simulink library "PB_Library_Master_Working"  (R2021a)
settings: Solver=VariableStepAuto  StartTime=0.0  StopTime=10.0  RelTol=1e-3
undefined symbols (not defined in the file): A_M, B_M, component_degradation_input, E0_M, f_sw, f_sw_M_aDF, flux_m_aDF, Fsw_M_aDF, insert, K_M, L_M_aDF, L_M_adf, P_Fe_Nom_aDF, Q_M, Q_rr, r_c, r_D, R_M, R_s_aDF, resistance_aDF, S_nom_aDF, SOC_Init_M, TFall_M_aDF, TRise_M_aDF, Trr_M_aDF, u_ce0, u_D0
libraries: $bdroot x76, Lib_Dyn_StateSpace_EMTAT x6, Lib_PF_BusLoadDC_TMATS x3, PB_Library_Master x3, simulink x3, TemperatureBlock x1
(part 3 of 5)

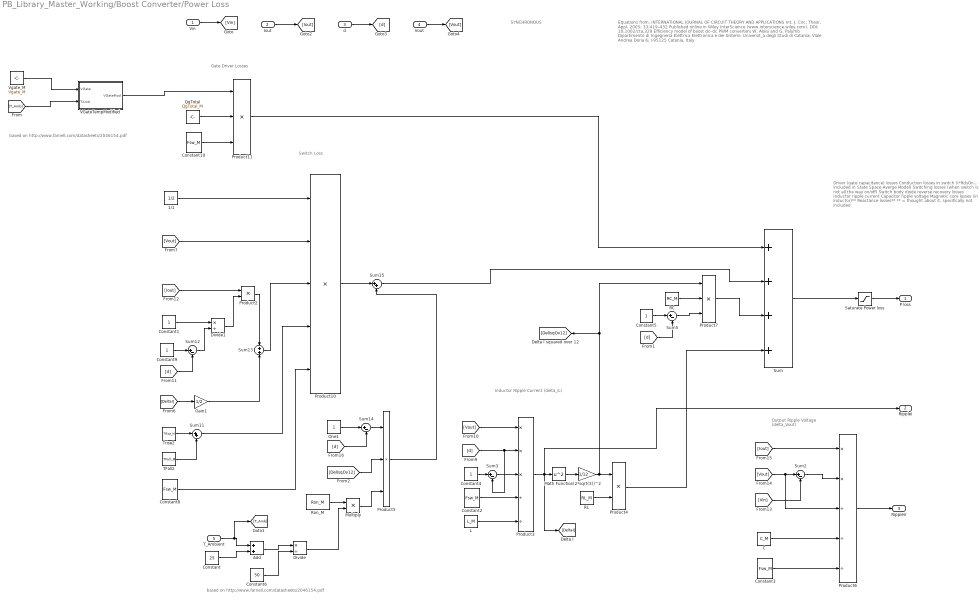
== system PB_Library_Master_Working/Boost Converter/Power Loss  ==
  note: Gate Driver Losses
  note: Output Ripple Voltage
      | (delta_Vout)
  note: Inductor Ripple Current
      | (delta_iL)
  note: Driver (gate capacitance) losses
      | Conduction losses in switch (I*RdsOn... included in State Space Averge Model)
      | Switching losses (when switch is not all the way on/off)
      | Switch body diode reverse recovery losses
      | Inductor ripple current
      | Capacitor ripple voltage
      | Magnetic core losses (in inductor)**
      | Reactance losses**
      | ** = thought about it, specifically not included
  note: SYNCHRONOUS
  note: Switch Loss
  note: Equations from:
      | INTERNATIONAL JOURNAL OF CIRCUIT THEORY AND APPLICATIONS
      | Int. J. Circ. Theor. Appl. 2005; 33:419–432
      | Published online in Wiley InterScience (www.interscience.wiley.com). DOI: 10.1002/cta.329
      | Efficiency model of boost dc–dc PWM converters
      | W. Aloisi and G. Palumb
      | Dipartimento di Ingegneria Elettrica Elettronica e dei Sistemi; Universit_a degli Studi di Catania;
      | Viale Andrea Doria 6; I-95125 Catania, Italy
  note: based on http://www.farnell.com/datasheets/2046154.pdf
  note: based on http://www.farnell.com/datasheets/2046154.pdf
  Vin : Inport
  Iout : Inport  Port=2
  d : Inport  Port=3
  Vout : Inport  Port=4
  "T_Ambient " : Inport  Port=5
  (2*sqrt(3))^2 : Gain  Gain=1/12
  1/1 : Constant  Value=1/2  VectorParams1D=off
  Add : Sum
  C : Constant  Value=C_M  VectorParams1D=off
  Constant : Constant  Value=25
  Constant{1,4..5,9} (4 alike) : Constant
  Constant{2..3,8,10} (4 alike) : Constant  Value=Fsw_M
  Constant6 : Constant  Value=50
  Divide : Product  Inputs=*/
  Divide1 : Product  Inputs=*/
  Gain1 : Gain  Gain=1/2
  L : Constant  Value=L_M  VectorParams1D=off
  Math Function : Math  Operator=square  SignedPower=on  SaturateOnIntegerOverflow=on
  Multiply : Product
  One1 : Constant  VectorParams1D=off
  Product10 : Product  Inputs=5
  Product11 : Product  Inputs=3
  Product2 : Product
  Product3 : Product  Inputs=***//
  Product4 : Product
  Product5 : Product  Inputs=3
  Product6 : Product  Inputs=**///
  Product7 : Product  Inputs=3
  QgTotal : Constant  Value=QgTotal_M  VectorParams1D=off
  RC : Constant  Value=RC_M  VectorParams1D=off
  RL : Constant  Value=RL_M  VectorParams1D=off
  Ron_M : Constant  Value=Ron_M
  Saturate Power loss : Saturate  UpperLimit=inf  LowerLimit=0
  Sum : Sum  Inputs=++++
  Sum11 : Sum  Inputs=|++
  Sum{2..3,5,12,14} (5 alike) : Sum  Inputs=|+-
  Sum13 : Sum
  Sum15 : Sum  Inputs=|++
  TFall2 : Constant  Value=TFall_M  VectorParams1D=off
  Trise2 : Constant  Value=TRise_M  VectorParams1D=off
  VGateTempModified : Subsystem
  "Vgate_M " : Constant  Value=Vgate_M
  " P loss" : Outport  VectorParamsAs1DForOutWhenUnconnected=off
  RippleI : Outport  Port=2  VectorParamsAs1DForOutWhenUnconnected=off
  RippleV : Outport  Port=3  VectorParamsAs1DForOutWhenUnconnected=off
  wires:
  VGateTempModified/1(VGateMod) -> Product11/1
  [T_Amb] -> VGateTempModified/2(TAmb)
  "Vgate_M "/1 -> VGateTempModified/1(VGate)
  Multiply/1 -> Product5/3
  Divide/1 -> Multiply/2
  Add/1 -> Divide/1
  Constant6/1 -> Divide/2
  Constant/1 -> Add/2
  "T_Ambient "/1 -> Add/1, [T_Amb]
  Sum15/1 -> Sum/2
  Product11/1 -> Sum/1
  Product7/1 -> Sum/3
  Product4/1 -> Sum/4
  QgTotal/1 -> Product11/2
  Constant10/1 -> Product11/3
  Product5/1 -> Sum15/2
  Product10/1 -> Sum15/1
  [DelIsqOv12] -> Product5/2
  Sum14/1 -> Product5/1
  Ron_M/1 -> Multiply/1
  One1/1 -> Sum14/1
  [d] -> Sum14/2
  Product6/1 -> RippleV/1
  Constant3/1 -> Product6/5
  C/1 -> Product6/4
  Sum2/1 -> Product6/2
  [Vin] -> Sum2/2
  [Vout] -> Sum2/1, Product6/3
  [Iout] -> Product6/1
  1/1/1 -> Product10/1
  [Vout] -> Product10/2
  Constant8/1 -> Product10/5
  Product2/1 -> Sum13/1
  Sum11/1 -> Product10/4
  Constant1/1 -> Divide1/1
  Trise2/1 -> Sum11/1
  TFall2/1 -> Sum11/2
  Divide1/1 -> Product2/2
  Sum12/1 -> Divide1/2
  Sum13/1 -> Product10/3
  Gain1/1 -> Sum13/2
  Constant9/1 -> Sum12/1
  [d] -> Sum12/2
  [DeltaI] -> Gain1/1
  [Iout] -> Product2/1
  Sum5/1 -> Product7/3
  [d] -> Sum5/2
  Constant5/1 -> Sum5/1
  Sum3/1 -> Product3/3
  Constant4/1 -> Sum3/1
  [Vout] -> Product3/1
  Constant2/1 -> Product3/4
  L/1 -> Product3/5
  Vout/1 -> [Vout]
  [d] -> Product3/2, Sum3/2
  d/1 -> [d]
  Iout/1 -> [Iout]
  Vin/1 -> [Vin]
  Sum/1 -> Saturate Power loss/1
  Saturate Power loss/1 -> " P loss"/1
  RL/1 -> Product4/2
  Product3/1 -> RippleI/1, Math Function/1, [DeltaI]
  (2*sqrt(3))^2/1 -> [DelIsqOv12], Product7/1, Product4/1
  Math Function/1 -> (2*sqrt(3))^2/1
  RC/1 -> Product7/2

== system PB_Library_Master_Working/Boost Converter/TempConv  ==
  Selected Input Units : Inport
  Unit Conversion : UnitConversion
  CelsiusOut : Outport  Unit=°C  VectorParamsAs1DForOutWhenUnconnected=off
  wires:
  Unit Conversion/1 -> CelsiusOut/1  "Celsius"
  Selected Input Units/1 -> Unit Conversion/1

== system PB_Library_Master_Working/Boost Converter Analytic/DC - DC Converter ==
  note: the aDF must decrease L_M
  note: Power B
  note: Current B
  note: Power B
  VIn : Inport
  x : Inport  Port=2
  d : Inport  Port=3
  dt : Inport  Port=4
  I_Demand : Inport  Port=5
  P loss : Inport  Port=6
  "T_Ambient " : Inport  Port=7
  " Dynamic State" : Subsystem  TreatAsAtomicUnit=on
  "1=dynamic, 0=static" : Display
  Add : Sum
  Bus Creator1 : BusCreator  Inputs=3
  Bus Creator3 : BusCreator  Inputs=3
  Bus Selector : BusSelector  OutputSignals=x,xdot,VB
  Constant : Constant  Value=[0, 1/C_M; -1/L_M, -(Ron_M+RC_M+RL_M)/L_M]  VectorParams1D=off
  Display : Display
  Divide : Product  Inputs=*/
  If : If
  MATLAB Function : MATLAB Function  TreatAsAtomicUnit=on
  Mux : Mux  Inputs=2
  Product3 : Product
  Steady State : Subsystem  TreatAsAtomicUnit=on
  Switch : Switch  Criteria=u2 ~= 0
  xdot : Constant  Value=zeros(2,1)  VectorParams1D=off
  VOut : Outport  VectorParamsAs1DForOutWhenUnconnected=off
  x_dot : Outport  Port=2  VectorParamsAs1DForOutWhenUnconnected=off
  x_new : Outport  Port=3  VectorParamsAs1DForOutWhenUnconnected=off
  I_Demanded : Outport  Port=4  VectorParamsAs1DForOutWhenUnconnected=off
  switchDyn : Outport  Port=5  VectorParamsAs1DForOutWhenUnconnected=off
  wires:
  "T_Ambient "/1 -> Steady State/3("T_Ambient "), Display/1
  Add/1 -> [PwrA]
  Mux/1 -> " Dynamic State"/2(u), Steady State/1(u)
  I_Demand/1 -> [IB], Mux/2
  [VA] -> Mux/1
  [x] -> x_new/1
  Bus Creator3/1 -> Switch/1
  Bus Selector/1 -> [x]  "<x>"
  Bus Selector/2 -> [xdot]  "<xdot>"
  Bus Selector/3 -> [VB]  "<VB>"
  xdot/1 -> Bus Creator1/2  "xdot"
  Steady State/2(VB) -> Bus Creator1/3  "VB"
  " Dynamic State"/1(xdot) -> Bus Creator3/2  "xdot"
  " Dynamic State"/2(VB) -> Bus Creator3/3  "VB"
  Switch/1 -> Bus Selector/1
  P loss/1 -> Add/2
  [PwrB] -> Add/1
  [xdot] -> x_dot/1
  d/1 -> " Dynamic State"/3(d), Steady State/2(d)
  x/1 -> " Dynamic State"/1(x), Bus Creator3/1  "x"
  Steady State/1(x) -> Bus Creator1/1  "x"
  dt/1 -> MATLAB Function/2(dt)
  If/2 -> Steady State/Action
  Constant/1 -> MATLAB Function/1(A1)
  If/1 -> " Dynamic State"/Action
  MATLAB Function/1(y) -> If/1, switchDyn/1, Switch/2, "1=dynamic, 0=static"/1
  [IA] -> I_Demanded/1
  [VA] -> Divide/2
  Divide/1 -> [IA]
  [PwrA] -> Divide/1
  [IB] -> Product3/2
  VIn/1 -> [VA]
  [VB] -> VOut/1  "V"
  Product3/1 -> [PwrB]
  [VB] -> Product3/1
  Bus Creator1/1 -> Switch/3

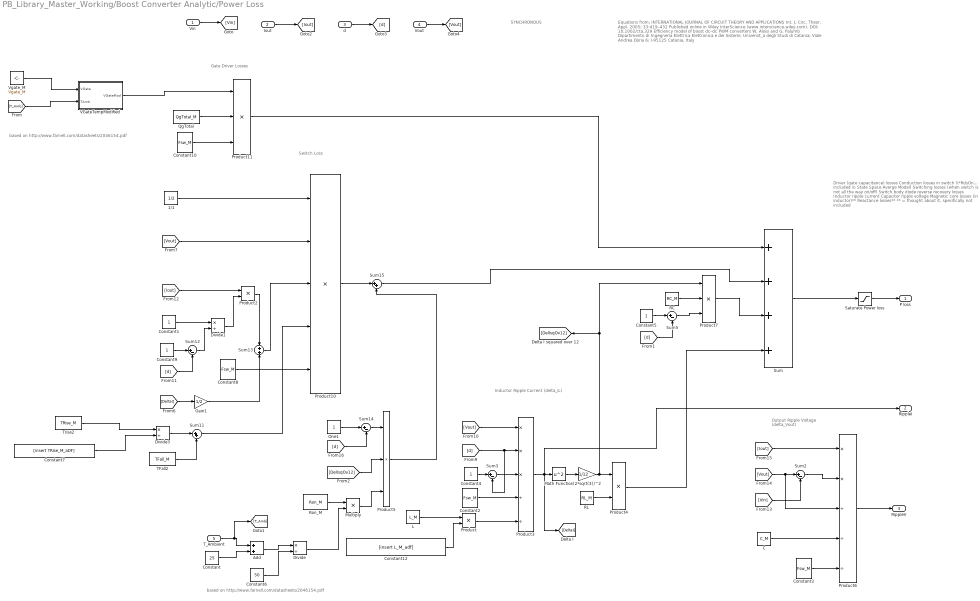
== system PB_Library_Master_Working/Boost Converter Analytic/Power Loss  ==
  note: Gate Driver Losses
  note: Output Ripple Voltage
      | (delta_Vout)
  note: Inductor Ripple Current
      | (delta_iL)
  note: Driver (gate capacitance) losses
      | Conduction losses in switch (I*RdsOn... included in State Space Averge Model)
      | Switching losses (when switch is not all the way on/off)
      | Switch body diode reverse recovery losses
      | Inductor ripple current
      | Capacitor ripple voltage
      | Magnetic core losses (in inductor)**
      | Reactance losses**
      | ** = thought about it, specifically not included
  note: SYNCHRONOUS
  note: Switch Loss
  note: Equations from:
      | INTERNATIONAL JOURNAL OF CIRCUIT THEORY AND APPLICATIONS
      | Int. J. Circ. Theor. Appl. 2005; 33:419–432
      | Published online in Wiley InterScience (www.interscience.wiley.com). DOI: 10.1002/cta.329
      | Efficiency model of boost dc–dc PWM converters
      | W. Aloisi and G. Palumb
      | Dipartimento di Ingegneria Elettrica Elettronica e dei Sistemi; Universit_a degli Studi di Catania;
      | Viale Andrea Doria 6; I-95125 Catania, Italy
  note: based on http://www.farnell.com/datasheets/2046154.pdf
  note: based on http://www.farnell.com/datasheets/2046154.pdf
  Vin : Inport
  Iout : Inport  Port=2
  d : Inport  Port=3
  Vout : Inport  Port=4
  "T_Ambient " : Inport  Port=5
  (2*sqrt(3))^2 : Gain  Gain=1/12
  1/1 : Constant  Value=1/2  VectorParams1D=off
  Add : Sum
  C : Constant  Value=C_M  VectorParams1D=off
  Constant : Constant  Value=25
  Constant{1,4..5,9} (4 alike) : Constant
  Constant{2..3,8,10} (4 alike) : Constant  Value=Fsw_M
  Constant12 : Constant  Value=[insert L_M_adf]
  Constant6 : Constant  Value=50
  Constant7 : Constant  Value=[insert TRise_M_aDF]
  Divide : Product  Inputs=*/
  Divide1 : Product  Inputs=*/
  Divide3 : Product  Inputs=*/
  Gain1 : Gain  Gain=1/2
  L : Constant  Value=L_M  VectorParams1D=off
  Math Function : Math  Operator=square  SignedPower=on  SaturateOnIntegerOverflow=on
  Multiply : Product
  One1 : Constant  VectorParams1D=off
  Product : Product
  Product10 : Product  Inputs=5
  Product11 : Product  Inputs=3
  Product2 : Product
  Product3 : Product  Inputs=***//
  Product4 : Product
  Product5 : Product  Inputs=3
  Product6 : Product  Inputs=**///
  Product7 : Product  Inputs=3
  QgTotal : Constant  Value=QgTotal_M  VectorParams1D=off
  RC : Constant  Value=RC_M  VectorParams1D=off
  RL : Constant  Value=RL_M  VectorParams1D=off
  Ron_M : Constant  Value=Ron_M
  Saturate Power loss : Saturate  UpperLimit=inf  LowerLimit=0
  Sum : Sum  Inputs=++++
  Sum11 : Sum  Inputs=|++
  Sum{2..3,5,12,14} (5 alike) : Sum  Inputs=|+-
  Sum13 : Sum
  Sum15 : Sum  Inputs=|++
  TFall2 : Constant  Value=TFall_M  VectorParams1D=off
  Trise2 : Constant  Value=TRise_M  VectorParams1D=off
  VGateTempModified : Subsystem
  "Vgate_M " : Constant  Value=Vgate_M
  " P loss" : Outport  VectorParamsAs1DForOutWhenUnconnected=off
  RippleI : Outport  Port=2  VectorParamsAs1DForOutWhenUnconnected=off
  RippleV : Outport  Port=3  VectorParamsAs1DForOutWhenUnconnected=off
  wires:
  VGateTempModified/1(VGateMod) -> Product11/1
  [T_Amb] -> VGateTempModified/2(TAmb)
  "Vgate_M "/1 -> VGateTempModified/1(VGate)
  Multiply/1 -> Product5/3
  Divide/1 -> Multiply/2
  Add/1 -> Divide/1
  Constant6/1 -> Divide/2
  Constant/1 -> Add/2
  "T_Ambient "/1 -> Add/1, [T_Amb]
  Sum15/1 -> Sum/2
  Product11/1 -> Sum/1
  Product7/1 -> Sum/3
  Product4/1 -> Sum/4
  QgTotal/1 -> Product11/2
  Product5/1 -> Sum15/2
  Product10/1 -> Sum15/1
  [DelIsqOv12] -> Product5/2
  Sum14/1 -> Product5/1
  One1/1 -> Sum14/1
  [d] -> Sum14/2
  Product6/1 -> RippleV/1
  C/1 -> Product6/4
  Sum2/1 -> Product6/2
  [Vin] -> Sum2/2
  [Vout] -> Sum2/1, Product6/3
  [Iout] -> Product6/1
  1/1/1 -> Product10/1
  [Vout] -> Product10/2
  Product2/1 -> Sum13/1
  Sum11/1 -> Product10/4
  Constant1/1 -> Divide1/1
  Divide1/1 -> Product2/2
  Sum12/1 -> Divide1/2
  Sum13/1 -> Product10/3
  Gain1/1 -> Sum13/2
  Constant9/1 -> Sum12/1
  [d] -> Sum12/2
  [DeltaI] -> Gain1/1
  [Iout] -> Product2/1
  Sum5/1 -> Product7/3
  [d] -> Sum5/2
  Constant5/1 -> Sum5/1
  Sum3/1 -> Product3/3
  Constant4/1 -> Sum3/1
  [Vout] -> Product3/1
  Vout/1 -> [Vout]
  [d] -> Product3/2, Sum3/2
  d/1 -> [d]
  Iout/1 -> [Iout]
  Vin/1 -> [Vin]
  Sum/1 -> Saturate Power loss/1
  Saturate Power loss/1 -> " P loss"/1
  RL/1 -> Product4/2
  Product3/1 -> RippleI/1, Math Function/1, [DeltaI]
  (2*sqrt(3))^2/1 -> [DelIsqOv12], Product7/1, Product4/1
  Math Function/1 -> (2*sqrt(3))^2/1
  RC/1 -> Product7/2
  Ron_M/1 -> Multiply/1
  Divide3/1 -> Sum11/1
  Trise2/1 -> Divide3/1
  Constant7/1 -> Divide3/2
  Constant10/1 -> Product11/3
  Constant8/1 -> Product10/5
  Constant2/1 -> Product3/4
  Constant3/1 -> Product6/5
  TFall2/1 -> Sum11/2
  Product/1 -> Product3/5
  L/1 -> Product/1
  Constant12/1 -> Product/2

== system PB_Library_Master_Working/Boost Converter Analytic/TempConv  ==
  Selected Input Units : Inport
  Unit Conversion : UnitConversion
  CelsiusOut : Outport  Unit=°C  VectorParamsAs1DForOutWhenUnconnected=off
  wires:
  Unit Conversion/1 -> CelsiusOut/1  "Celsius"
  Selected Input Units/1 -> Unit Conversion/1

== system PB_Library_Master_Working/Buck Converter/DC - DC Converter ==
  note: Power B
  note: Current B
  note: Power A
  NodeA : Inport
  IAg : Inport  Port=2
  x : Inport  Port=3
  d : Inport  Port=4
  dt : Inport  Port=5
  Iout : Inport  Port=6
  P loss : Inport  Port=7
  "T_Ambient " : Inport  Port=8
  " Dynamic State" : Subsystem  TreatAsAtomicUnit=on
  "1=dynamic, 0=static" : Display
  Add : Sum  Inputs=+-
  Bus Creator1 : BusCreator  Inputs=3
  Bus Creator3 : BusCreator  Inputs=3
  Bus Selector : BusSelector  OutputSignals=x,xdot,VB
  Constant : Constant  Value=[0, 1/C_M; -1/L_M, -(Ron_M+RC_M+RL_M)/L_M]  VectorParams1D=off
  Divide : Product  Commented=on  Inputs=*/
  Goto12 : Goto  Commented=on  GotoTag=IB
  Goto14 : From  Commented=on  GotoTag=PwrB
  Goto15 : From  Commented=on  GotoTag=VB
  Goto5 : From  Commented=on  GotoTag=IB
  If : If
  MATLAB Function : MATLAB Function  TreatAsAtomicUnit=on
  Mux : Mux  Inputs=2
  Negate : Gain  Commented=through  Gain=-1
  Product3 : Product
  Steady State : Subsystem  TreatAsAtomicUnit=on
  Switch : Switch  Criteria=u2 ~= 0
  xdot : Constant  Value=zeros(2,1)  VectorParams1D=off
  NodeB : Outport  VectorParamsAs1DForOutWhenUnconnected=off
  x_dot : Outport  Port=2  VectorParamsAs1DForOutWhenUnconnected=off
  x_new : Outport  Port=3  VectorParamsAs1DForOutWhenUnconnected=off
  PElec : Outport  Port=4  VectorParamsAs1DForOutWhenUnconnected=off
  IA : Outport  Port=5  VectorParamsAs1DForOutWhenUnconnected=off
  switchDyn : Outport  Port=6  VectorParamsAs1DForOutWhenUnconnected=off
  wires:
  "T_Ambient "/1 -> Steady State/3("T_Ambient ")
  Negate/1 -> [PwrB]
  Mux/1 -> " Dynamic State"/2(u), Steady State/1(u)
  Iout/1 -> Mux/2
  [VA] -> Mux/1
  [x] -> x_new/1
  Bus Creator3/1 -> Switch/1
  Bus Selector/1 -> [x]  "<x>"
  Bus Selector/2 -> [xdot]  "<xdot>"
  Bus Selector/3 -> [VB]  "<VB>"
  xdot/1 -> Bus Creator1/2  "xdot"
  Steady State/2(VB) -> Bus Creator1/3  "VB"
  " Dynamic State"/1(xdot) -> Bus Creator3/2  "xdot"
  " Dynamic State"/2(VB) -> Bus Creator3/3  "VB"
  Switch/1 -> Bus Selector/1
  Add/1 -> Negate/1
  P loss/1 -> Add/2
  [PwrA] -> Add/1
  [xdot] -> x_dot/1
  d/1 -> " Dynamic State"/3(d), Steady State/2(d)
  x/1 -> " Dynamic State"/1(x), Bus Creator3/1  "x"
  Steady State/1(x) -> Bus Creator1/1  "x"
  dt/1 -> MATLAB Function/2(dt)
  If/2 -> Steady State/Action
  Constant/1 -> MATLAB Function/1(A1)
  If/1 -> " Dynamic State"/Action
  MATLAB Function/1(y) -> If/1, switchDyn/1, Switch/2, "1=dynamic, 0=static"/1
  [IA] -> IA/1
  Goto5/1 -> ?  "I"
  IAg/1 -> [IA]
  Goto15/1 -> Divide/2
  Divide/1 -> Goto12/1
  Goto14/1 -> Divide/1
  [IA] -> Product3/2
  NodeA/1 -> [VA]
  [VB] -> NodeB/1  "V"
  Product3/1 -> [PwrA]
  [VA] -> Product3/1
  Bus Creator1/1 -> Switch/3
  [PwrB] -> PElec/1

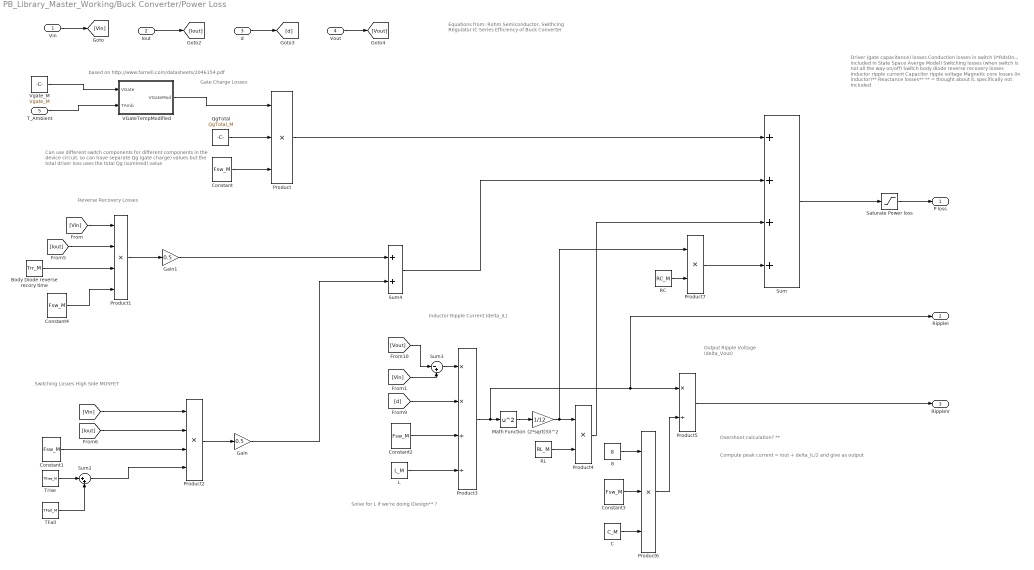
== system PB_Library_Master_Working/Buck Converter/Power Loss  ==
  note: based on http://www.farnell.com/datasheets/2046154.pdf
  note: Overshoot calculation? **
  note: Output Ripple Voltage
      | (delta_Vout)
  note: Inductor Ripple Current
      | (delta_iL)
  note: Reverse Recovery Losses
  note: Switching Losses High Side MOSFET
  note: Driver (gate capacitance) losses
      | Conduction losses in switch (I*RdsOn... included in State Space Averge Model)
      | Switching losses (when switch is not all the way on/off)
      | Switch body diode reverse recovery losses
      | Inductor ripple current
      | Capacitor ripple voltage
      | Magnetic core losses (in inductor)**
      | Reactance losses**
      | ** = thought about it, specifically not included
  note: Can use different switch components for different components in
      | the device circuit, so can have separate Qg (gate charge) values
      | but the total driver loss uses the total Qg (summed) value
  note: Gate Charge Losses
  note: Solve for L if we're doing iDesign** ?
  note: Compute peak current = Iout + delta_IL/2 and give as output
  note: Equations from:
      | Rohm Semiconductor, Swithcing Regulator IC Series
      | Efficiency of Buck Converter
  Vin : Inport
  Iout : Inport  Port=2
  d : Inport  Port=3
  Vout : Inport  Port=4
  "T_Ambient " : Inport  Port=5
  (2*sqrt(3))^2 : Gain  Gain=1/12
  8 : Constant  Value=8  VectorParams1D=off
  Body Diode reverse recory time : Constant  Value=Trr_M  VectorParams1D=off
  C : Constant  Value=C_M  VectorParams1D=off
  Constant{,1..4} (5 alike) : Constant  Value=Fsw_M
  Gain : Gain  Gain=0.5
  Gain1 : Gain  Gain=0.5
  L : Constant  Value=L_M  VectorParams1D=off
  Math Function : Math  Operator=square  SignedPower=on  SaturateOnIntegerOverflow=on
  Product : Product  Inputs=3
  Product1 : Product  Inputs=4
  Product2 : Product  Inputs=4
  Product3 : Product  Inputs=**//
  Product4 : Product
  Product5 : Product  Inputs=*/
  Product6 : Product  Inputs=3
  Product7 : Product
  QgTotal : Constant  Value=QgTotal_M  VectorParams1D=off
  RC : Constant  Value=RC_M  VectorParams1D=off
  RL : Constant  Value=RL_M  VectorParams1D=off
  Saturate Power loss : Saturate  UpperLimit=inf  LowerLimit=0
  Sum : Sum  Inputs=++++
  Sum2 : Sum  Inputs=|++
  Sum3 : Sum  Inputs=|-+
  Sum4 : Sum
  TFall : Constant  Value=TFall_M  VectorParams1D=off
  Trise : Constant  Value=TRise_M  VectorParams1D=off
  VGateTempModified : Subsystem
  Vgate_M : Constant  Value=Vgate_M
  " P loss" : Outport  VectorParamsAs1DForOutWhenUnconnected=off
  RippleI : Outport  Port=2  VectorParamsAs1DForOutWhenUnconnected=off
  RippleV : Outport  Port=3  VectorParamsAs1DForOutWhenUnconnected=off
  wires:
  VGateTempModified/1("VGateMod ") -> Product/1
  "T_Ambient "/1 -> VGateTempModified/2(TAmb)
  Vgate_M/1 -> VGateTempModified/1("VGate ")
  Gain1/1 -> Sum4/1
  Product1/1 -> Gain1/1
  Constant4/1 -> Product1/4
  Body Diode reverse recory time/1 -> Product1/3
  [Iout] -> Product1/2
  [Vin] -> Product1/1
  Gain/1 -> Sum4/2
  Product2/1 -> Gain/1
  Constant3/1 -> Product6/2
  Constant2/1 -> Product3/3
  Constant1/1 -> Product2/3
  Constant/1 -> Product/3
  [Vout] -> Sum3/1
  Vout/1 -> [Vout]
  [d] -> Product3/2
  d/1 -> [d]
  [Iout] -> Product2/2
  Iout/1 -> [Iout]
  [Vin] -> Sum3/2
  [Vin] -> Product2/1
  Vin/1 -> [Vin]
  Sum/1 -> Saturate Power loss/1
  Saturate Power loss/1 -> " P loss"/1
  QgTotal/1 -> Product/2
  Sum4/1 -> Sum/2
  Trise/1 -> Sum2/1
  TFall/1 -> Sum2/2
  Product/1 -> Sum/1
  Sum2/1 -> Product2/4
  Sum3/1 -> Product3/1
  L/1 -> Product3/4
  Product4/1 -> Sum/3
  RL/1 -> Product4/2
  Product3/1 -> Product5/1, RippleI/1, Math Function/1
  (2*sqrt(3))^2/1 -> Product7/1, Product4/1
  Math Function/1 -> (2*sqrt(3))^2/1
  Product6/1 -> Product5/2
  8/1 -> Product6/1
  C/1 -> Product6/3
  Product5/1 -> RippleV/1
  RC/1 -> Product7/2
  Product7/1 -> Sum/4

== system PB_Library_Master_Working/Buck Converter/TempConv  ==
  Selected Input Units : Inport
  Unit Conversion : UnitConversion
  CelsiusOut : Outport  Unit=°C  VectorParamsAs1DForOutWhenUnconnected=off
  wires:
  Unit Conversion/1 -> CelsiusOut/1  "Celsius"
  Selected Input Units/1 -> Unit Conversion/1

== system PB_Library_Master_Working/Buck Converter Analytic/DC - DC Converter ==
  note: Power A
  note: Current A
  note: Power B
  VIn : Inport
  x : Inport  Port=2
  d : Inport  Port=3
  dt : Inport  Port=4
  I_Demand : Inport  Port=5
  P loss : Inport  Port=6
  "T_Ambient " : Inport  Port=7
  " Dynamic State" : Subsystem  TreatAsAtomicUnit=on
  "1=dynamic, 0=static" : Display
  Add : Sum
  Bus Creator1 : BusCreator  Inputs=3
  Bus Creator3 : BusCreator  Inputs=3
  Bus Selector : BusSelector  OutputSignals=x,xdot,VB
  Constant : Constant  Value=[0, 1/C_M; -1/L_M, -(Ron_M+RC_M+RL_M)/L_M]  VectorParams1D=off
  Divide : Product  Inputs=*/
  If : If
  MATLAB Function : MATLAB Function  TreatAsAtomicUnit=on
  Mux : Mux  Inputs=2
  Product3 : Product
  Steady State : Subsystem  TreatAsAtomicUnit=on
  Switch : Switch  Criteria=u2 ~= 0
  xdot : Constant  Value=zeros(2,1)  VectorParams1D=off
  Vout : Outport  VectorParamsAs1DForOutWhenUnconnected=off
  x_dot : Outport  Port=2  VectorParamsAs1DForOutWhenUnconnected=off
  x_new : Outport  Port=3  VectorParamsAs1DForOutWhenUnconnected=off
  I_Demanded : Outport  Port=4  VectorParamsAs1DForOutWhenUnconnected=off
  switchDyn : Outport  Port=5  VectorParamsAs1DForOutWhenUnconnected=off
  wires:
  Bus Creator1/1 -> Switch/3
  [VB] -> Vout/1  "V"
  VIn/1 -> [VA]
  [IB] -> Product3/2
  [IA] -> I_Demanded/1
  MATLAB Function/1(y) -> "1=dynamic, 0=static"/1, Switch/2, switchDyn/1, If/1
  If/1 -> " Dynamic State"/Action
  Constant/1 -> MATLAB Function/1(A1)
  If/2 -> Steady State/Action
  dt/1 -> MATLAB Function/2(dt)
  Steady State/1(x) -> Bus Creator1/1  "x"
  x/1 -> Bus Creator3/1, " Dynamic State"/1(x)  "x"
  d/1 -> Steady State/2(d), " Dynamic State"/3(d)
  [xdot] -> x_dot/1
  P loss/1 -> Add/2
  Switch/1 -> Bus Selector/1
  " Dynamic State"/2(VB) -> Bus Creator3/3  "VB"
  " Dynamic State"/1(xdot) -> Bus Creator3/2  "xdot"
  Steady State/2(VB) -> Bus Creator1/3  "VB"
  xdot/1 -> Bus Creator1/2  "xdot"
  Bus Selector/3 -> [VB]  "<VB>"
  Bus Selector/2 -> [xdot]  "<xdot>"
  Bus Selector/1 -> [x]  "<x>"
  Bus Creator3/1 -> Switch/1
  [x] -> x_new/1
  [VA] -> Mux/1
  Mux/1 -> Steady State/1(u), " Dynamic State"/2(u)
  "T_Ambient "/1 -> Steady State/3("T_Ambient ")
  I_Demand/1 -> [IB], Mux/2
  [VB] -> Product3/1  "V"
  Product3/1 -> [PwrB]
  Divide/1 -> [IA]
  [PwrB] -> Add/1
  Add/1 -> [PwrA]
  [PwrA] -> Divide/1
  [VA] -> Divide/2

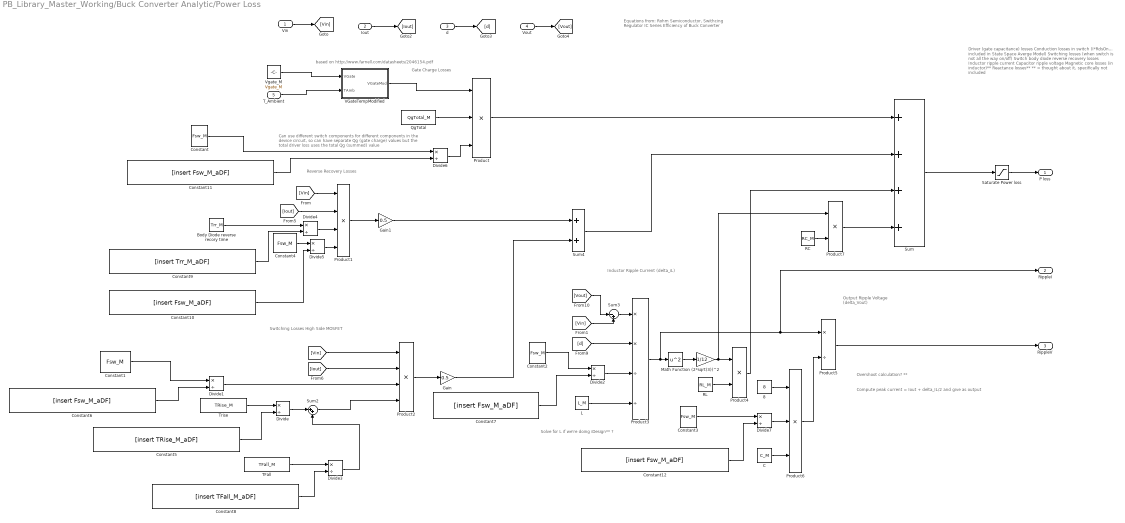
== system PB_Library_Master_Working/Buck Converter Analytic/Power Loss  ==
  note: Equations from:
      | Rohm Semiconductor, Swithcing Regulator IC Series
      | Efficiency of Buck Converter
  note: Compute peak current = Iout + delta_IL/2 and give as output
  note: Solve for L if we're doing iDesign** ?
  note: Gate Charge Losses
  note: Can use different switch components for different components in
      | the device circuit, so can have separate Qg (gate charge) values
      | but the total driver loss uses the total Qg (summed) value
  note: Driver (gate capacitance) losses
      | Conduction losses in switch (I*RdsOn... included in State Space Averge Model)
      | Switching losses (when switch is not all the way on/off)
      | Switch body diode reverse recovery losses
      | Inductor ripple current
      | Capacitor ripple voltage
      | Magnetic core losses (in inductor)**
      | Reactance losses**
      | ** = thought about it, specifically not included
  note: Switching Losses High Side MOSFET
  note: Reverse Recovery Losses
  note: Inductor Ripple Current
      | (delta_iL)
  note: Output Ripple Voltage
      | (delta_Vout)
  note: Overshoot calculation? **
  note: based on http://www.farnell.com/datasheets/2046154.pdf
  Vin : Inport
  Iout : Inport  Port=2
  d : Inport  Port=3
  Vout : Inport  Port=4
  "T_Ambient " : Inport  Port=5
  (2*sqrt(3))^2 : Gain  Gain=1/12
  8 : Constant  Value=8  VectorParams1D=off
  Body Diode reverse recory time : Constant  Value=Trr_M  VectorParams1D=off
  C : Constant  Value=C_M  VectorParams1D=off
  Constant{,1..4} (5 alike) : Constant  Value=Fsw_M
  Constant{6..7,10..12} (5 alike) : Constant  Value=[insert Fsw_M_aDF]
  Constant5 : Constant  Value=[insert TRise_M_aDF]
  Constant8 : Constant  Value=[insert TFall_M_aDF]
  Constant9 : Constant  Value=[insert Trr_M_aDF]
  Divide{,1..7} (8 alike) : Product  Inputs=*/
  Gain : Gain  Gain=0.5
  Gain1 : Gain  Gain=0.5
  L : Constant  Value=L_M  VectorParams1D=off
  Math Function : Math  Operator=square  SignedPower=on  SaturateOnIntegerOverflow=on
  Product : Product  Inputs=3
  Product1 : Product  Inputs=4
  Product2 : Product  Inputs=4
  Product3 : Product  Inputs=**//
  Product4 : Product
  Product5 : Product  Inputs=*/
  Product6 : Product  Inputs=3
  Product7 : Product
  QgTotal : Constant  Value=QgTotal_M  VectorParams1D=off
  RC : Constant  Value=RC_M  VectorParams1D=off
  RL : Constant  Value=RL_M  VectorParams1D=off
  Saturate Power loss : Saturate  UpperLimit=inf  LowerLimit=0
  Sum : Sum  Inputs=++++
  Sum2 : Sum  Inputs=|++
  Sum3 : Sum  Inputs=|-+
  Sum4 : Sum
  TFall : Constant  Value=TFall_M  VectorParams1D=off
  Trise : Constant  Value=TRise_M  VectorParams1D=off
  VGateTempModified : Subsystem
  Vgate_M : Constant  Value=Vgate_M
  " P loss" : Outport  VectorParamsAs1DForOutWhenUnconnected=off
  RippleI : Outport  Port=2  VectorParamsAs1DForOutWhenUnconnected=off
  RippleV : Outport  Port=3  VectorParamsAs1DForOutWhenUnconnected=off
  wires:
  Product7/1 -> Sum/4
  RC/1 -> Product7/2
  Product5/1 -> RippleV/1
  C/1 -> Product6/3
  8/1 -> Product6/1
  Product6/1 -> Product5/2
  Math Function/1 -> (2*sqrt(3))^2/1
  (2*sqrt(3))^2/1 -> Product4/1, Product7/1
  Product3/1 -> Math Function/1, RippleI/1, Product5/1
  RL/1 -> Product4/2
  Product4/1 -> Sum/3
  L/1 -> Product3/4
  Sum3/1 -> Product3/1
  Sum2/1 -> Product2/4
  Product/1 -> Sum/1
  Sum4/1 -> Sum/2
  QgTotal/1 -> Product/2
  Saturate Power loss/1 -> " P loss"/1
  Sum/1 -> Saturate Power loss/1
  Vin/1 -> [Vin]
  [Vin] -> Product2/1
  [Vin] -> Sum3/2
  Iout/1 -> [Iout]
  [Iout] -> Product2/2
  d/1 -> [d]
  [d] -> Product3/2
  Vout/1 -> [Vout]
  [Vout] -> Sum3/1
  Product2/1 -> Gain/1
  Gain/1 -> Sum4/2
  [Vin] -> Product1/1
  [Iout] -> Product1/2
  Product1/1 -> Gain1/1
  Gain1/1 -> Sum4/1
  Vgate_M/1 -> VGateTempModified/1("VGate ")
  "T_Ambient "/1 -> VGateTempModified/2(TAmb)
  VGateTempModified/1("VGateMod ") -> Product/1
  Divide/1 -> Sum2/1
  Trise/1 -> Divide/1
  Constant5/1 -> Divide/2
  Divide1/1 -> Product2/3
  Constant1/1 -> Divide1/1
  Constant6/1 -> Divide1/2
  Divide2/1 -> Product3/3
  Constant2/1 -> Divide2/1
  Constant7/1 -> Divide2/2
  Divide3/1 -> Sum2/2
  TFall/1 -> Divide3/1
  Constant8/1 -> Divide3/2
  Divide4/1 -> Product1/3
  Body Diode reverse recory time/1 -> Divide4/1
  Constant9/1 -> Divide4/2
  Divide5/1 -> Product1/4
  Constant4/1 -> Divide5/1
  Constant10/1 -> Divide5/2
  Divide6/1 -> Product/3
  Constant/1 -> Divide6/1
  Constant11/1 -> Divide6/2
  Divide7/1 -> Product6/2
  Constant3/1 -> Divide7/1
  Constant12/1 -> Divide7/2

== system PB_Library_Master_Working/Buck Converter Analytic/TempConv  ==
  Selected Input Units : Inport
  Unit Conversion : UnitConversion
  CelsiusOut : Outport  Unit=°C  VectorParamsAs1DForOutWhenUnconnected=off
  wires:
  Selected Input Units/1 -> Unit Conversion/1
  Unit Conversion/1 -> CelsiusOut/1  "Celsius"

== system PB_Library_Master_Working/Electrothermal_Battery_Model/Battery Core (w// Q) ==
  it_base : Inport
  IgIn : Inport  Port=2
  Tavg : Inport  Port=3
  BatteryCore : Subsystem
  Constant1 : Constant  Value=SOC_Init_M
  Vout : Outport  VectorParamsAs1DForOutWhenUnconnected=off
  SOC : Outport  Port=2  VectorParamsAs1DForOutWhenUnconnected=off
  it : Outport  Port=3  VectorParamsAs1DForOutWhenUnconnected=off
  Heat_Generated : Outport  Port=4  VectorParamsAs1DForOutWhenUnconnected=off
  wires:
  IgIn/1 -> BatteryCore/3("Battery Current (A) ")
  Constant1/1 -> BatteryCore/1("SOC Init (%) ")
  Tavg/1 -> BatteryCore/4("Tavg ")
  it_base/1 -> BatteryCore/2("it base (Ah) ")
  BatteryCore/2(it (Ah)) -> it/1
  BatteryCore/1(Battery Voltage (V)) -> Vout/1
  BatteryCore/3(SOC (%)) -> SOC/1
  BatteryCore/4(Heat_Generated) -> Heat_Generated/1

== system PB_Library_Master_Working/Electrothermal_Battery_Model/TempConv  ==
  Selected Input Units : Inport
  Unit Conversion : UnitConversion
  CelsiusOut : Outport  Unit=°C  VectorParamsAs1DForOutWhenUnconnected=off
  wires:
  Unit Conversion/1 -> CelsiusOut/1  "Celsius"
  Selected Input Units/1 -> Unit Conversion/1

== system PB_Library_Master_Working/Electrothermal_Battery_Model/it_Dot = f(i) ==
  i : Inport
  Convert As/s to Ah/s : Gain  Gain=1/3600
  it_Dot : Outport  VectorParamsAs1DForOutWhenUnconnected=off
  wires:
  Convert As/s to Ah/s/1 -> it_Dot/1
  i/1 -> Convert As/s to Ah/s/1

== system PB_Library_Master_Working/Electrothermal_Battery_Model_Analytic/Battery Core (w// Q) ==
  it_base : Inport
  I_Demand : Inport  Port=2
  Tavg : Inport  Port=3
  BatteryCore : Subsystem
  Constant1 : Constant  Value=SOC_Init_M
  Vout : Outport  VectorParamsAs1DForOutWhenUnconnected=off
  SOC : Outport  Port=2  VectorParamsAs1DForOutWhenUnconnected=off
  it : Outport  Port=3  VectorParamsAs1DForOutWhenUnconnected=off
  Heat_Generated : Outport  Port=4  VectorParamsAs1DForOutWhenUnconnected=off
  wires:
  I_Demand/1 -> BatteryCore/3("Battery Current (A) ")
  Constant1/1 -> BatteryCore/1("SOC Init (%) ")
  Tavg/1 -> BatteryCore/4("Tavg ")
  it_base/1 -> BatteryCore/2("it base (Ah) ")
  BatteryCore/2(it (Ah)) -> it/1
  BatteryCore/1(Battery Voltage (V)) -> Vout/1
  BatteryCore/3(SOC (%)) -> SOC/1
  BatteryCore/4(Heat_Generated) -> Heat_Generated/1

== system PB_Library_Master_Working/Electrothermal_Battery_Model_Analytic/it_Dot = f(i) ==
  i : Inport
  Convert As/s to Ah/s : Gain  Gain=1/3600
  it_Dot : Outport  VectorParamsAs1DForOutWhenUnconnected=off
  wires:
  Convert As/s to Ah/s/1 -> it_Dot/1
  i/1 -> Convert As/s to Ah/s/1

== system PB_Library_Master_Working/Generator/Copper Losses ==
  Iq : Inport
  Id1 : Inport  Port=2
  Constant : Constant  Value=[insert R_s_aDF]
  Constant1 : Constant  Value=[insert R_s_aDF]
  Divide : Product  Inputs=/*
  Divide1 : Product  Inputs=*/
  Gain1 : Gain  Gain=R_s
  Gain2 : Gain  Gain=R_s
  Square1 : Math  Operator=square  SignedPower=on  SaturateOnIntegerOverflow=on
  Square2 : Math  Operator=square  SignedPower=on  SaturateOnIntegerOverflow=on
  Sum : Sum
  P_Cu : Outport  VectorParamsAs1DForOutWhenUnconnected=off
  wires:
  Sum/1 -> P_Cu/1
  Square1/1 -> Gain1/1
  Iq/1 -> Square1/1
  Divide1/1 -> Sum/2
  Divide/1 -> Sum/1
  Gain1/1 -> Divide1/1
  Constant1/1 -> Divide1/2
  Gain2/1 -> Divide/2
  Id1/1 -> Square2/1
  Square2/1 -> Gain2/1
  Constant/1 -> Divide/1

== system PB_Library_Master_Working/Generator/Field Weakening and d current  ==
  note: Needs: S_n,flux_m,L_s
  S : Inport
  Constant : Constant  Value=flux_m
  Constant1 : Constant  Value=S_nom
  Constant2 : Constant  Value=[insert flux_m_aDF]
  Divide : Product  Inputs=*/
  Gain : Gain  Gain=1/L_s
  Product : Product
  Product1 : Product
  Subtract : Sum  Inputs=+-
  Switch : Switch  Criteria=u2 > Threshold  Threshold=S_nom
  flux_s : Outport  VectorParamsAs1DForOutWhenUnconnected=off
  Id : Outport  Port=2  VectorParamsAs1DForOutWhenUnconnected=off
  wires:
  S/1 -> Divide/2, Switch/2
  Product/1 -> Switch/1
  Divide/1 -> Product/2
  Switch/1 -> Subtract/1, flux_s/1
  Subtract/1 -> Gain/1
  Gain/1 -> Id/1
  Product1/1 -> Switch/3, Product/1, Subtract/2
  Constant/1 -> Product1/1
  Constant2/1 -> Product1/2
  Constant1/1 -> Divide/1

== system PB_Library_Master_Working/Generator/I_rms (Actual) ==
  note: I_RMS (actual) = sqrt(Id^2 + Iq^2)
  iq : Inport
  id : Inport  Port=2
  Isign : Inport  Port=3
  Add : Sum
  Mult : Product  Inputs=**
  Square : Math  Operator=square  SaturateOnIntegerOverflow=on
  Square Root : Sqrt  SaturateOnIntegerOverflow=on
  Square1 : Math  Operator=square  SaturateOnIntegerOverflow=on
  to RMS : Gain  Gain=1/sqrt(3)
  Is : Outport
  wires:
  Add/1 -> Square Root/1
  Square/1 -> Add/1
  Mult/1 -> to RMS/1
  Isign/1 -> Mult/1
  to RMS/1 -> Is/1  "Is"
  Square Root/1 -> Mult/2
  iq/1 -> Square1/1
  Square1/1 -> Add/2
  id/1 -> Square/1

== system PB_Library_Master_Working/Generator/Iq ==
  Is : Inport
  Id : Inport  Port=2
  Add1 : Sum  Inputs=+-
  Square Root1 : Sqrt  SaturateOnIntegerOverflow=on
  Square2 : Math  Operator=square  SignedPower=on  SaturateOnIntegerOverflow=on
  Square3 : Math  Operator=square  SignedPower=on  SaturateOnIntegerOverflow=on
  Iq : Outport  VectorParamsAs1DForOutWhenUnconnected=off
  wires:
  Is/1 -> Square2/1
  Id/1 -> Square3/1
  Square2/1 -> Add1/1
  Square3/1 -> Add1/2
  Add1/1 -> Square Root1/1
  Square Root1/1 -> Iq/1

== system PB_Library_Master_Working/Generator/Iron Loss ==
  w_elec : Inport
  Constant : Constant  Value=S_nom*((2*pi)/60)*pp
  Constant1 : Constant  Value=[insert P_Fe_Nom_aDF]
  Divide : Product  Inputs=*/
  Divide1 : Product  Inputs=*/
  Gain : Gain  Gain=P_Fe_Nom
  P_Fe : Outport  VectorParamsAs1DForOutWhenUnconnected=off
  wires:
  Divide/1 -> Gain/1
  w_elec/1 -> Divide/1
  Divide1/1 -> P_Fe/1
  Constant1/1 -> Divide1/2
  Constant/1 -> Divide/2
  Gain/1 -> Divide1/1

== system PB_Library_Master_Working/Generator/Power Factor Calc ==
  Id : Inport
  Iq : Inport  Port=2
  Vd : Inport  Port=3
  Vq : Inport  Port=4
  P : Inport  Port=5
  Divide : Product  Inputs=*/
  Product : Product
  Product1 : Product
  Subtract : Sum  Inputs=+-
  Trigonometric Function : Trigonometry  Operator=atan
  Out1 : Outport  VectorParamsAs1DForOutWhenUnconnected=off
  wires:
  Trigonometric Function/1 -> Out1/1
  Divide/1 -> Trigonometric Function/1
  P/1 -> Divide/2
  Subtract/1 -> Divide/1
  Product/1 -> Subtract/1
  Product1/1 -> Subtract/2
  Iq/1 -> Product1/2
  Vd/1 -> Product1/1
  Id/1 -> Product/2
  Vq/1 -> Product/1

== system PB_Library_Master_Working/Generator/Torque Saturation Logic ==
  note: Needs: P_m_max, T_ref_max
  T_ref_in : Inport
  S : Inport  Port=2
  Constant1 : Constant  Value=P_out_max
  Divide : Product  Inputs=*/
  Product : Product
  Sat (ft-lbs) : Saturate  UpperLimit=T_nom*1.3558  LowerLimit=0
  Switch : Switch  Criteria=u2 > Threshold  Threshold=P_out_max
  T_ref_sat : Outport  VectorParamsAs1DForOutWhenUnconnected=off
  wires:
  T_ref_in/1 -> Sat (ft-lbs)/1, Product/1  "Nm"
  Constant1/1 -> Divide/1  "W"
  S/1 -> Product/2, Divide/2
  Product/1 -> Switch/2  "W"
  Divide/1 -> Switch/1  "Nm"
  Switch/1 -> T_ref_sat/1
  Sat (ft-lbs)/1 -> Switch/3  "Nm"

== system PB_Library_Master_Working/Generator/Vdq ==
  Id : Inport
  w_elec : Inport  Port=2
  Iq : Inport  Port=3
  Constant : Constant  Value=[insert R_s_aDF]
  Constant1 : Constant  Value=[insert flux_m_aDF]
  Constant2 : Constant  Value=[insert R_s_aDF]
  Divide : Product  Inputs=*/
  Divide1 : Product  Inputs=/*
  Gain : Gain  Gain=R_s
  Gain1 : Gain  Gain=R_s
  Gain2 : Gain  Gain=L_s
  Gain3 : Gain  Gain=flux_m
  Product : Product
  Product1 : Product
  Product2 : Product
  Subtract : Sum  Inputs=+-
  Sum : Sum  Inputs=+++
  Vd : Outport  VectorParamsAs1DForOutWhenUnconnected=off
  Vq : Outport  Port=2  VectorParamsAs1DForOutWhenUnconnected=off
  wires:
  Id/1 -> Gain/1, Product1/1
  Iq/1 -> Gain1/1, Product/2
  w_elec/1 -> Gain2/1, Gain3/1
  Gain2/1 -> Product/1, Product1/2
  Product/1 -> Subtract/2
  Subtract/1 -> Vd/1
  Product1/1 -> Sum/1
  Sum/1 -> Vq/1
  Product2/1 -> Sum/3
  Gain3/1 -> Product2/1
  Divide/1 -> Sum/2
  Gain1/1 -> Divide/1
  Divide1/1 -> Subtract/1
  Constant1/1 -> Product2/2
  Gain/1 -> Divide1/2
  Constant/1 -> Divide/2
  Constant2/1 -> Divide1/1

== system PB_Library_Master_Working/Generator/Vs ==
  Vd : Inport
  Vq : Inport  Port=2
  Add : Sum
  Square : Math  Operator=square  SignedPower=on  SaturateOnIntegerOverflow=on
  Square Root : Sqrt  SaturateOnIntegerOverflow=on
  Square1 : Math  Operator=square  SignedPower=on  SaturateOnIntegerOverflow=on
  Vs : Outport  VectorParamsAs1DForOutWhenUnconnected=off
  wires:
  Square Root/1 -> Vs/1
  Add/1 -> Square Root/1
  Square/1 -> Add/2
  Square1/1 -> Add/1
  Vd/1 -> Square1/1
  Vq/1 -> Square/1

== system PB_Library_Master_Working/Inverter/Diode Conduction Losses ==
  note: the aDF must decrease u_D_M
  note: You need to read from graphs:
      |
      | -U_ce0
      | -Rc=dU_ce/dI_c (linear)
      | -U_D0
      | -R_D=dU_D/dI_D (linear)
  I_M : Inport
  PF : Inport  Port=2
  m : Inport  Port=3
  T : Inport  Port=4
  1-D Lookup Table r_D : Lookup_n-D  NumberOfTableDimensions=1  BreakpointsForDimension1=T_M  Table=R_D_M  InternalRulePriority=Speed  RndMeth=Simplest  InputSameDT=on
  1-D Lookup Table u_D0 : Lookup_n-D  NumberOfTableDimensions=1  BreakpointsForDimension1=T_M  Table=u_D_M  InternalRulePriority=Speed  RndMeth=Simplest  InputSameDT=on
  Constant : Constant  Value=1/(2*pi)
  Constant1 : Constant  Value=1/8
  Gain : Gain  Commented=on  Gain=u_D0
  Gain1 : Gain  Gain=1/8
  Gain2 : Gain  Commented=on  Gain=r_D
  Gain3 : Gain  Gain=1/(3*pi)
  Product{,1..4} (5 alike) : Product
  Square : Math  Operator=square  SignedPower=on  SaturateOnIntegerOverflow=on
  Sum : Sum  Inputs=+-
  Sum2 : Sum
  Sum3 : Sum  Inputs=-+
  P_CD : Outport  VectorParamsAs1DForOutWhenUnconnected=off
  wires:
  Product/1 -> Sum2/1
  Product2/1 -> Sum2/2
  Sum2/1 -> P_CD/1
  I_M/1 -> Product3/1  "I_M"
  Product3/1 -> Product/2, Square/1
  Constant/1 -> Sum/1
  PF/1 -> Product1/1
  m/1 -> Product1/2
  Gain1/1 -> Sum/2
  Product1/1 -> Gain3/1, Gain1/1
  Sum/1 -> Product/1
  Square/1 -> Product4/1
  Gain3/1 -> Sum3/1
  Product4/1 -> Product2/1
  Constant1/1 -> Sum3/2
  Sum3/1 -> Product2/2
  T/1 -> 1-D Lookup Table u_D0/1, 1-D Lookup Table r_D/1
  1-D Lookup Table u_D0/1 -> Product3/2
  1-D Lookup Table r_D/1 -> Product4/2

== system PB_Library_Master_Working/Inverter/Diode Switching Losses ==
  note: I_Drrpeak=2Qrr/trr
  note: Worst case - voltage across diode is supply voltage
  Input : Inport
  Constant1 : Constant  Value=f_sw
  Gain : Gain  Gain=.25*Q_rr
  Product2 : Product
  P_rec_D : Outport  VectorParamsAs1DForOutWhenUnconnected=off
  wires:
  Product2/1 -> P_rec_D/1
  Constant1/1 -> Product2/2  "I_M"
  Gain/1 -> Product2/1
  Input/1 -> Gain/1  "V_batt"

== system PB_Library_Master_Working/Inverter/IGBT Conduction Losses ==
  note: You need to read from graphs:
      |
      | -U_ce0
      | -Rc=dU_ce/dI_c (linear)
      | -U_D0
      | -R_D=dU_D/dI_D (linear)
  I_M : Inport
  PF : Inport  Port=2
  m : Inport  Port=3
  T : Inport  Port=4
  1-D Lookup Table r_c : Lookup_n-D  NumberOfTableDimensions=1  BreakpointsForDimension1=T_M  Table=R_c_M  InternalRulePriority=Speed  RndMeth=Simplest  InputSameDT=on
  1-D Lookup Table u_ce0 : Lookup_n-D  NumberOfTableDimensions=1  BreakpointsForDimension1=T_M  Table=u_ce0_M  InternalRulePriority=Speed  RndMeth=Simplest  InputSameDT=on
  Constant : Constant  Value=1/(2*pi)
  Constant1 : Constant  Value=1/8
  Gain : Gain  Commented=on  Gain=u_ce0
  Gain1 : Gain  Gain=1/8
  Gain2 : Gain  Commented=on  Gain=r_c
  Gain3 : Gain  Gain=1/(3*pi)
  Product{,1..4} (5 alike) : Product
  Square : Math  Operator=square  SignedPower=on  SaturateOnIntegerOverflow=on
  Sum : Sum
  Sum2 : Sum
  Sum3 : Sum
  P_CT : Outport  VectorParamsAs1DForOutWhenUnconnected=off
  wires:
  Product/1 -> Sum2/1
  Product2/1 -> Sum2/2
  Sum2/1 -> P_CT/1
  I_M/1 -> Product3/1  "I_M"
  Product3/1 -> Product/2, Square/1
  Constant/1 -> Sum/1
  PF/1 -> Product1/1
  m/1 -> Product1/2
  Gain1/1 -> Sum/2
  Product1/1 -> Gain3/1, Gain1/1
  Sum/1 -> Product/1
  Square/1 -> Product4/1
  Gain3/1 -> Sum3/1
  Product4/1 -> Product2/1
  Constant1/1 -> Sum3/2
  Sum3/1 -> Product2/2
  T/1 -> 1-D Lookup Table u_ce0/1, 1-D Lookup Table r_c/1
  1-D Lookup Table u_ce0/1 -> Product3/2
  1-D Lookup Table r_c/1 -> Product4/2

== system PB_Library_Master_Working/Inverter/IGBT Switching Losses ==
  note: the aDF must increase E1_M
  I_ce : Inport
  T : Inport  Port=2
  1-D Lookup Table E0 : Lookup_n-D  NumberOfTableDimensions=1  BreakpointsForDimension1=T_M  Table=E0_M  InternalRulePriority=Speed  RndMeth=Simplest  InputSameDT=on
  1-D Lookup Table E1 : Lookup_n-D  NumberOfTableDimensions=1  BreakpointsForDimension1=T_M  Table=E1_M  InternalRulePriority=Speed  RndMeth=Simplest  InputSameDT=on
  Add : Sum
  Constant : Constant  Value=f_sw_M
  Constant1 : Constant  Value=[insert f_sw_M_aDF]
  Divide : Product  Inputs=*/
  Product : Product
  Product1 : Product
  P_ST : Outport  VectorParamsAs1DForOutWhenUnconnected=off
  wires:
  Product/1 -> P_ST/1
  Add/1 -> Product/1
  I_ce/1 -> Product1/1
  1-D Lookup Table E0/1 -> Add/1
  Product1/1 -> Add/2
  T/1 -> 1-D Lookup Table E0/1, 1-D Lookup Table E1/1
  1-D Lookup Table E1/1 -> Product1/2
  Divide/1 -> Product/2
  Constant/1 -> Divide/1
  Constant1/1 -> Divide/2

== system PB_Library_Master_Working/Inverter/I_Ripple ==
  V_batt : Inport
  "V_M " : Inport  Port=2
  Constant : Constant  Value=L_s_M
  Constant1 : Constant  Value=[insert f_sw_M_aDF]
  Divide : Product  Inputs=*/
  Divide1 : Product  Inputs=*/
  Gain : Gain  Gain=sqrt(2)
  Gain1 : Gain  Gain=2
  Gain2 : Gain  Gain=f_sw_M
  Product : Product
  Product1 : Product
  Subtract : Sum  Inputs=+-
  Inport Value : Outport  VectorParamsAs1DForOutWhenUnconnected=off
  wires:
  "V_M "/1 -> Product/2, Gain/1
  Gain/1 -> Subtract/2
  V_batt/1 -> Subtract/1, Product1/1
  Subtract/1 -> Product/1
  Product/1 -> Divide/1
  Constant/1 -> Gain1/1
  Gain1/1 -> Product1/2
  Product1/1 -> Gain2/1
  Divide/1 -> Inport Value/1
  Divide1/1 -> Divide/2
  Gain2/1 -> Divide1/1
  Constant1/1 -> Divide1/2

== system PB_Library_Master_Working/Inverter/P_in_mot ==
  V_s : Inport
  I : Inport  Port=2
  PF : Inport  Port=3
  Gain : Gain  Gain=sqrt(3)
  Product : Product  Inputs=3
  P_in_mot : Outport  VectorParamsAs1DForOutWhenUnconnected=off
  wires:
  I/1 -> Product/2
  PF/1 -> Product/3
  V_s/1 -> Product/1
  Gain/1 -> P_in_mot/1
  Product/1 -> Gain/1

== system PB_Library_Master_Working/Inverter/mVal ==
  V_s : Inport
  V_batt : Inport  Port=2
  Divide : Product  Inputs=*/
  Gain : Gain  Gain=sqrt(2)
  m : Outport  VectorParamsAs1DForOutWhenUnconnected=off
  V_batt_pass : Outport  Port=2  VectorParamsAs1DForOutWhenUnconnected=off
  wires:
  Divide/1 -> m/1
  V_s/1 -> Gain/1
  Gain/1 -> Divide/1
  V_batt/1 -> V_batt_pass/1, Divide/2

== system PB_Library_Master_Working/Motor/Copper Losses ==
  Id : Inport
  Iq : Inport  Port=2
  Constant : Constant  Value=[insert R_s_aDF]
  Constant1 : Constant  Value=[insert R_s_aDF]
  Divide : Product  Inputs=*/
  Divide1 : Product  Inputs=/*
  Gain : Gain  Gain=R_s
  Gain1 : Gain  Gain=R_s
  Square : Math  Operator=square  SignedPower=on  SaturateOnIntegerOverflow=on
  Square1 : Math  Operator=square  SignedPower=on  SaturateOnIntegerOverflow=on
  Sum : Sum
  P_Cu : Outport  VectorParamsAs1DForOutWhenUnconnected=off
  wires:
  Iq/1 -> Square1/1
  Id/1 -> Square/1
  Square/1 -> Gain/1
  Square1/1 -> Gain1/1
  Sum/1 -> P_Cu/1
  Gain1/1 -> Divide/1
  Constant/1 -> Divide/2
  Gain/1 -> Divide1/2
  Divide1/1 -> Sum/1
  Divide/1 -> Sum/2
  Constant1/1 -> Divide1/1

== system PB_Library_Master_Working/Motor/Field Weakening and d current  ==
  note: the aDF needs to decrease S_nom
  note: Needs: S_n,flux_m,L_s
  S : Inport
  Constant : Constant  Value=flux_m
  Constant1 : Constant  Value=S_nom
  Constant2 : Constant  Value=[insert flux_m_aDF]
  Constant3 : Constant  Value=[insert S_nom_aDF]
  Divide : Product  Inputs=*/
  Gain : Gain  Gain=1/L_s
  Product : Product
  Product1 : Product
  Product2 : Product
  Subtract : Sum  Inputs=+-
  Switch : Switch  Criteria=u2 > Threshold  Threshold=S_nom*mot_ans.S_nom_aDF.Data(end)
  flux_s : Outport  VectorParamsAs1DForOutWhenUnconnected=off
  id : Outport  Port=2  VectorParamsAs1DForOutWhenUnconnected=off
  wires:
  S/1 -> Divide/2, Switch/2
  Product/1 -> Switch/1
  Divide/1 -> Product/2
  Switch/1 -> Subtract/1, flux_s/1
  Subtract/1 -> Gain/1
  Gain/1 -> id/1
  Constant/1 -> Product1/1
  Product1/1 -> Subtract/2, Product/1, Switch/3
  Constant2/1 -> Product1/2
  Product2/1 -> Divide/1
  Constant1/1 -> Product2/1
  Constant3/1 -> Product2/2

== system PB_Library_Master_Working/Motor/Iron Loss ==
  w_elec : Inport
  Constant : Constant  Value=S_nom*((2*pi)/60)*pp
  Constant1 : Constant  Value=[insert P_Fe_Nom_aDF]
  Constant2 : Constant  Value=[insert S_nom_aDF]
  Divide : Product  Inputs=*/
  Divide1 : Product  Inputs=*/
  Gain : Gain  Gain=P_Fe_Nom
  Product : Product
  P_Fe : Outport  VectorParamsAs1DForOutWhenUnconnected=off
  wires:
  w_elec/1 -> Divide/1
  Divide/1 -> Gain/1
  Gain/1 -> Divide1/1
  Divide1/1 -> P_Fe/1
  Constant1/1 -> Divide1/2
  Product/1 -> Divide/2
  Constant/1 -> Product/1
  Constant2/1 -> Product/2

== system PB_Library_Master_Working/Motor/Is ==
  Id : Inport
  Iq : Inport  Port=2
  Add : Sum
  Square : Math  Operator=square  SignedPower=on  SaturateOnIntegerOverflow=on
  Square Root : Sqrt  SaturateOnIntegerOverflow=on
  Square1 : Math  Operator=square  SignedPower=on  SaturateOnIntegerOverflow=on
  Is : Outport  VectorParamsAs1DForOutWhenUnconnected=off
  wires:
  Iq/1 -> Square/1
  Id/1 -> Square1/1
  Square1/1 -> Add/1
  Square/1 -> Add/2
  Add/1 -> Square Root/1
  Square Root/1 -> Is/1

== system PB_Library_Master_Working/Motor/Power Factor Calc  ==
  Id : Inport
  Iq : Inport  Port=2
  Vd : Inport  Port=3
  Vq : Inport  Port=4
  P : Inport  Port=5
  Display : Display
  Divide : Product  Inputs=*/
  Product : Product
  Product1 : Product
  Subtract : Sum  Inputs=+-
  Trigonometric Function : Trigonometry  Operator=atan
  Out1 : Outport  VectorParamsAs1DForOutWhenUnconnected=off
  wires:
  Vq/1 -> Product/1
  Id/1 -> Product/2
  Vd/1 -> Product1/1
  Iq/1 -> Product1/2
  Product1/1 -> Subtract/2
  Product/1 -> Subtract/1
  Subtract/1 -> Divide/1
  P/1 -> Divide/2, Display/1
  Divide/1 -> Trigonometric Function/1
  Trigonometric Function/1 -> Out1/1

== system PB_Library_Master_Working/Motor/Torque Saturation Logic ==
  note: Needs: P_m_max, T_ref_max
  T_ref_in : Inport
  S : Inport  Port=2
  Constant1 : Constant  Value=P_out_max
  Divide : Product  Inputs=*/
  Product : Product
  Sat in ft-lbs : Saturate  UpperLimit=T_nom  LowerLimit=0
  Switch : Switch  Criteria=u2 > Threshold  Threshold=P_out_max
  ft-lbs to Nm : Gain  Gain=1.3558
  ft-lbs to Nm1 : Gain  Gain=1.3558
  T_ref_sat : Outport  VectorParamsAs1DForOutWhenUnconnected=off
  wires:
  T_ref_in/1 -> Sat in ft-lbs/1, ft-lbs to Nm/1  "ft-lbs"
  Constant1/1 -> Divide/1  "W"
  S/1 -> Product/2, Divide/2
  Sat in ft-lbs/1 -> ft-lbs to Nm1/1
  Product/1 -> Switch/2  "W"
  Divide/1 -> Switch/1  "Nm"
  Switch/1 -> T_ref_sat/1
  ft-lbs to Nm/1 -> Product/1
  ft-lbs to Nm1/1 -> Switch/3  "Nm"

== system PB_Library_Master_Working/Motor/Vdq ==
  Id : Inport
  w_elec : Inport  Port=2
  Iq : Inport  Port=3
  Constant : Constant  Value=[insert flux_m_aDF]
  Constant1 : Constant  Value=[insert R_s_aDF]
  Constant2 : Constant  Value=[insert R_s_aDF]
  Divide : Product  Inputs=/*
  Divide1 : Product  Inputs=*/
  Gain : Gain  Gain=R_s
  Gain1 : Gain  Gain=R_s
  Gain2 : Gain  Gain=L_s
  Gain3 : Gain  Gain=flux_m
  Product : Product
  Product1 : Product
  Product2 : Product
  Subtract : Sum  Inputs=+-
  Sum : Sum  Inputs=+++
  Vd : Outport  VectorParamsAs1DForOutWhenUnconnected=off
  Vq : Outport  Port=2  VectorParamsAs1DForOutWhenUnconnected=off
  wires:
  Id/1 -> Product1/1, Gain/1
  Iq/1 -> Gain1/1, Product/2
  w_elec/1 -> Gain3/1, Gain2/1
  Gain2/1 -> Product/1, Product1/2
  Product/1 -> Subtract/2
  Subtract/1 -> Vd/1
  Product1/1 -> Sum/1
  Sum/1 -> Vq/1
  Gain3/1 -> Product2/1
  Product2/1 -> Sum/3
  Constant/1 -> Product2/2
  Divide/1 -> Subtract/1
  Gain/1 -> Divide/2
  Constant1/1 -> Divide/1
  Divide1/1 -> Sum/2
  Gain1/1 -> Divide1/1
  Constant2/1 -> Divide1/2

== system PB_Library_Master_Working/Motor/Vs ==
  Vd : Inport
  Vq : Inport  Port=2
  Add : Sum
  Square : Math  Operator=square  SignedPower=on  SaturateOnIntegerOverflow=on
  Square Root : Sqrt  SaturateOnIntegerOverflow=on
  Square1 : Math  Operator=square  SignedPower=on  SaturateOnIntegerOverflow=on
  Vs : Outport  VectorParamsAs1DForOutWhenUnconnected=off
  wires:
  Vq/1 -> Square/1
  Vd/1 -> Square1/1
  Square1/1 -> Add/1
  Square/1 -> Add/2
  Add/1 -> Square Root/1
  Square Root/1 -> Vs/1

== system PB_Library_Master_Working/Rectifier/Diode Conduction Losses1 ==
  note: the aDF must increase u_D_M
  note: You need to read from graphs:
      |
      | -U_ce0
      | -Rc=dU_ce/dI_c (linear)
      | -U_D0
      | -R_D=dU_D/dI_D (linear)
  I_M : Inport
  PF : Inport  Port=2
  m : Inport  Port=3
  T : Inport  Port=4
  1-D Lookup Table r_D : Lookup_n-D  NumberOfTableDimensions=1  BreakpointsForDimension1=T_M  Table=R_D_M  InternalRulePriority=Speed  RndMeth=Simplest  InputSameDT=on
  1-D Lookup Table u_D0 : Lookup_n-D  NumberOfTableDimensions=1  BreakpointsForDimension1=T_M  Table=u_D_M/rect_ans.u_D_M_aDF.Data(end)  InternalRulePriority=Speed  RndMeth=Simplest  InputSameDT=on
  Constant : Constant  Value=1/(2*pi)
  Constant1 : Constant  Value=1/8
  Gain : Gain  Commented=on  Gain=u_D0
  Gain1 : Gain  Gain=1/8
  Gain2 : Gain  Commented=on  Gain=r_D
  Gain3 : Gain  Gain=1/(3*pi)
  Product{,1..4} (5 alike) : Product
  Square : Math  Operator=square  SignedPower=on  SaturateOnIntegerOverflow=on
  Sum : Sum  Inputs=+-
  Sum2 : Sum
  Sum3 : Sum  Inputs=-+
  P_CD : Outport  VectorParamsAs1DForOutWhenUnconnected=off
  wires:
  1-D Lookup Table r_D/1 -> Product4/2
  1-D Lookup Table u_D0/1 -> Product3/2
  T/1 -> 1-D Lookup Table r_D/1, 1-D Lookup Table u_D0/1
  Sum3/1 -> Product2/2
  Constant1/1 -> Sum3/2
  Product4/1 -> Product2/1
  Gain3/1 -> Sum3/1
  Square/1 -> Product4/1
  Sum/1 -> Product/1
  Product1/1 -> Gain1/1, Gain3/1
  Gain1/1 -> Sum/2
  m/1 -> Product1/2
  PF/1 -> Product1/1
  Constant/1 -> Sum/1
  Product3/1 -> Square/1, Product/2
  I_M/1 -> Product3/1  "I_M"
  Sum2/1 -> P_CD/1
  Product2/1 -> Sum2/2
  Product/1 -> Sum2/1
